simulink model "es_own"  (Simulink 7.6)
settings: Solver=ode45  StartTime=0.0  StopTime=5  MaxStep=0.01  RelTol=1e-3
values from neighbouring files (symbols this model uses):
  x0 = [-1; -1]    [es6driver.m]
libraries: simulink x1
settings Model: Creator=patrizio  LastModifiedBy=patrizio

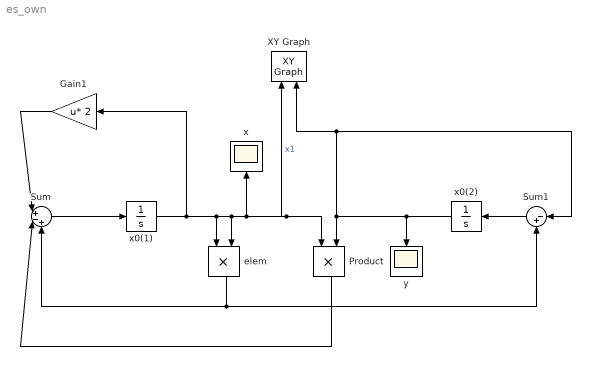
== system es_own ==
  Gain1 : Gain  Gain=2  Multiplication=Matrix(u*K)
  Product : Product  RndMeth=Zero
  Sum : Sum  Inputs=|+-+
  Sum1 : Sum  Inputs=|-+
  XY Graph : simulink/Sinks/XY Graph  SystemSampleTime=-1  xmin=-20  xmax=20  ymin=-20  ymax=20  st=-1
  "elem " : Product  RndMeth=Zero
  x : Scope
  x0(1) : Integrator  InitialCondition=x0(1)
  x0(2) : Integrator  InitialCondition=x0(2)
  y : Scope
  wires:
  x0(1)/1 -> Gain1/1, "elem "/1, "elem "/2, Product/1, XY Graph/1, x/1  "x1"
  x0(2)/1 -> Product/2, XY Graph/2, Sum1/1, y/1
  Product/1 -> Sum/2
  Sum1/1 -> x0(2)/1
  Sum/1 -> x0(1)/1
  "elem "/1 -> Sum/3, Sum1/2
  Gain1/1 -> Sum/1
